simulink model "pvtest1"  (R2022b)
settings: Solver=ode45  StartTime=0.0  StopTime=100.0  RelTol=1e-3
values from neighbouring files (symbols this model uses):
  Ki1 = double(1)    [untitled.m]
  Ki2 = double(1)    [untitled.m]
  Kp1 = double(1)    [untitled.m]
  Kp2 = double(1)    [untitled.m]
undefined symbols (not defined in the file or in its folder): Kd1, Kd2, magnitude
libraries: slpidlib x2
settings Model: Creator=19693  LastModifiedBy=TT

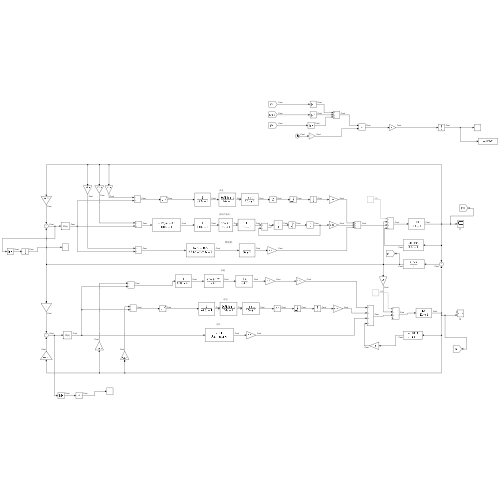
[thumbnail: Simulink's stored preview of the top-level diagram]
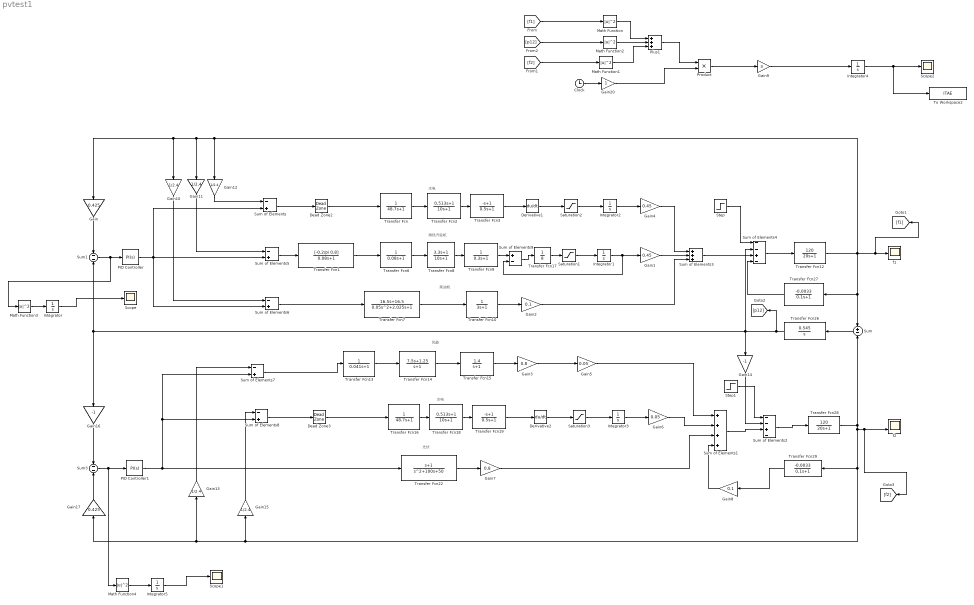
== system pvtest1 ==
  note: 光伏
  note: 风能
  note: 柴油机
  note: 再热汽轮机
  note: 水电
  note: 水电
  Clock : Clock
  Dead Zone2 : DeadZone  LowerValue=-0.0002  UpperValue=0.0002
  Dead Zone3 : DeadZone  LowerValue=-0.0002  UpperValue=0.0002
  Derivative1 : Derivative
  Derivative2 : Derivative
  Gain : Gain  Gain=0.425
  Gain1 : Gain  Gain=0.45
  Gain{10..13,15} (5 alike) : Gain  Gain=1/2.4
  Gain14 : Gain  Gain=-1
  Gain16 : Gain  Gain=-1
  Gain17 : Gain  Gain=0.425
  Gain2 : Gain  Gain=0.1
  Gain20 : Gain
  Gain3 : Gain  Gain=0.8
  Gain4 : Gain  Gain=0.45
  Gain5 : Gain  Gain=0.05
  Gain6 : Gain  Gain=0.05
  Gain7 : Gain  Gain=0.8
  Gain8 : Gain  Gain=0.1
  Gain9 : Gain  Gain=3
  Integrator{,1..5} (6 alike) : Integrator
  Math Function{,1..4} (5 alike) : Math  Operator=magnitude^2
  PID Controller : slpidlib/PID Controller  Controller=PI  Form=Parallel  TimeDomain=Continuous-time  UseExternalTs=off  SampleTime=-1  IntegratorMethod=Forward Euler  FilterMethod=Forward Euler  ControllerParametersSource=internal  P=Kp1  I=Ki1  UseKiTs=off  D=Kd1  N=100  UseFilter=on  TunerSelectOption=Transfer Function Based (PID Tuner App)  InitialConditionSource=internal  InitialConditionForIntegrator=0  InitialConditionForFilter=0  DifferentiatorICPrevScaledInput=0  ExternalReset=none  TrackingMode=off  Kt=1  LimitOutput=off  SatLimitsSource=internal  UpperSaturationLimit=inf  LowerSaturationLimit=-inf  LinearizeAsGain=on  AntiWindupMode=none  Kb=1  LimitIntegrator=off  UpperIntegratorSaturationLimit=inf  LowerIntegratorSaturationLimit=-inf  POutMin=[]  POutMax=[]  IOutMin=[]  IOutMax=[]  DOutMin=[]  DOutMax=[]  NOutMin=[]  NOutMax=[]  SumOutMin=[]  SumOutMax=[]  SaturationOutMin=[]  SaturationOutMax=[]  PParamMin=[]  PParamMax=[]  IParamMin=[]  IParamMax=[]  DParamMin=[]  DParamMax=[]  NParamMin=[]  NParamMax=[]  KbParamMin=[]  KbParamMax=[]  KtParamMin=[]  KtParamMax=[]  KbOutMin=[]  KbOutMax=[]  KtOutMin=[]  KtOutMax=[]  IntegratorOutMin=[]  IntegratorOutMax=[]  FilterOutMin=[]  FilterOutMax=[]  SumI1OutMin=[]  SumI1OutMax=[]  SumI2OutMin=[]  SumI2OutMax=[]  SumI3OutMin=[]  SumI3OutMax=[]  SumI4OutMin=[]  SumI4OutMax=[]  SumDOutMin=[]  SumDOutMax=[]  DifferentiatorOutMin=[]  DifferentiatorOutMax=[]  FilterDiffOutCoefMin=[]  FilterDiffOutCoefMax=[]  ReciprocalOutMin=[]  ReciprocalOutMax=[]  SumDenOutMin=[]  SumDenOutMax=[]  SumNumOutMin=[]  SumNumOutMax=[]  DivideOutMin=[]  DivideOutMax=[]  UdiffTsProdOutMin=[]  UdiffTsProdOutMax=[]  NTsProdOutMin=[]  NTsProdOutMax=[]  UintegralTsProdOutMin=[]  UintegralTsProdOutMax=[]  UngainTsProdOutMin=[]  UngainTsProdOutMax=[]  ClampingZeroOutDataTypeStr=Inherit: Inherit via back propagation  ClampingZeroOutMin=[]  ClampingZeroOutMax=[]  FilterDenConstantOutDataTypeStr=Inherit: Inherit via back propagation  FilterDenConstantOutMin=[]  FilterDenConstantOutMax=[]  PCopyOutDataTypeStr=Inherit: Inherit via back propagation  PCopyOutMin=[]  PCopyOutMax=[]  NCopyOutDataTypeStr=Inherit: Inherit via back propagation  NCopyOutMin=[]  NCopyOutMax=[]  IntegratorContinuousStateAttributes=''  IntegratorStateMustResolveToSignalObject=off  IntegratorRTWStateStorageClass=Auto  FilterContinuousStateAttributes=''  FilterStateMustResolveToSignalObject=off  FilterRTWStateStorageClass=Auto  ParallelPVariant=InternalParameters  IdealPVariant=Disabled  IVariant=InternalParameters  DVariant=Disabled  IntegratorVariant=Continuous  SatVariant=Disabled  AWVariant=Passthrough  PCopyVariant=Disabled  TRVariant=Disabled  FdbkBlocksVariant=Forward  IdealPFdbkVariant=Disabled  SatFdbkVariant=Disabled  DerivativeFilterVariant=Disabled  NVariant=Disabled  NCopyVariant=Disabled_SignalSpec  FilterICVariant=Disabled  IntegratorICVariant=InternalICs  ExternalResetVariant=Disabled  TRSumVariant=Passthrough  SumFdbkVariant=Disabled  SumVariant=Sum_PI  TsampFilterVariant=InternalTs  TsampNgainVariant=Passthrough  TsampIntegralVariant=Passthrough  ExternalSaturationOutDataTypeStr=Inherit: Same as second input
  PID Controller1 : slpidlib/PID Controller  Controller=PI  Form=Parallel  TimeDomain=Continuous-time  UseExternalTs=off  SampleTime=-1  IntegratorMethod=Forward Euler  FilterMethod=Forward Euler  ControllerParametersSource=internal  P=Kp2  I=Ki2  UseKiTs=off  D=Kd2  N=100  UseFilter=on  TunerSelectOption=Transfer Function Based (PID Tuner App)  InitialConditionSource=internal  InitialConditionForIntegrator=0  InitialConditionForFilter=0  DifferentiatorICPrevScaledInput=0  ExternalReset=none  TrackingMode=off  Kt=1  LimitOutput=off  SatLimitsSource=internal  UpperSaturationLimit=inf  LowerSaturationLimit=-inf  LinearizeAsGain=on  AntiWindupMode=none  Kb=1  LimitIntegrator=off  UpperIntegratorSaturationLimit=inf  LowerIntegratorSaturationLimit=-inf  POutMin=[]  POutMax=[]  IOutMin=[]  IOutMax=[]  DOutMin=[]  DOutMax=[]  NOutMin=[]  NOutMax=[]  SumOutMin=[]  SumOutMax=[]  SaturationOutMin=[]  SaturationOutMax=[]  PParamMin=[]  PParamMax=[]  IParamMin=[]  IParamMax=[]  DParamMin=[]  DParamMax=[]  NParamMin=[]  NParamMax=[]  KbParamMin=[]  KbParamMax=[]  KtParamMin=[]  KtParamMax=[]  KbOutMin=[]  KbOutMax=[]  KtOutMin=[]  KtOutMax=[]  IntegratorOutMin=[]  IntegratorOutMax=[]  FilterOutMin=[]  FilterOutMax=[]  SumI1OutMin=[]  SumI1OutMax=[]  SumI2OutMin=[]  SumI2OutMax=[]  SumI3OutMin=[]  SumI3OutMax=[]  SumI4OutMin=[]  SumI4OutMax=[]  SumDOutMin=[]  SumDOutMax=[]  DifferentiatorOutMin=[]  DifferentiatorOutMax=[]  FilterDiffOutCoefMin=[]  FilterDiffOutCoefMax=[]  ReciprocalOutMin=[]  ReciprocalOutMax=[]  SumDenOutMin=[]  SumDenOutMax=[]  SumNumOutMin=[]  SumNumOutMax=[]  DivideOutMin=[]  DivideOutMax=[]  UdiffTsProdOutMin=[]  UdiffTsProdOutMax=[]  NTsProdOutMin=[]  NTsProdOutMax=[]  UintegralTsProdOutMin=[]  UintegralTsProdOutMax=[]  UngainTsProdOutMin=[]  UngainTsProdOutMax=[]  ClampingZeroOutDataTypeStr=Inherit: Inherit via back propagation  ClampingZeroOutMin=[]  ClampingZeroOutMax=[]  FilterDenConstantOutDataTypeStr=Inherit: Inherit via back propagation  FilterDenConstantOutMin=[]  FilterDenConstantOutMax=[]  PCopyOutDataTypeStr=Inherit: Inherit via back propagation  PCopyOutMin=[]  PCopyOutMax=[]  NCopyOutDataTypeStr=Inherit: Inherit via back propagation  NCopyOutMin=[]  NCopyOutMax=[]  IntegratorContinuousStateAttributes=''  IntegratorStateMustResolveToSignalObject=off  IntegratorRTWStateStorageClass=Auto  FilterContinuousStateAttributes=''  FilterStateMustResolveToSignalObject=off  FilterRTWStateStorageClass=Auto  ParallelPVariant=InternalParameters  IdealPVariant=Disabled  IVariant=InternalParameters  DVariant=Disabled  IntegratorVariant=Continuous  SatVariant=Disabled  AWVariant=Passthrough  PCopyVariant=Disabled  TRVariant=Disabled  FdbkBlocksVariant=Forward  IdealPFdbkVariant=Disabled  SatFdbkVariant=Disabled  DerivativeFilterVariant=Disabled  NVariant=Disabled  NCopyVariant=Disabled_SignalSpec  FilterICVariant=Disabled  IntegratorICVariant=InternalICs  ExternalResetVariant=Disabled  TRSumVariant=Passthrough  SumFdbkVariant=Disabled  SumVariant=Sum_PI  TsampFilterVariant=InternalTs  TsampNgainVariant=Passthrough  TsampIntegralVariant=Passthrough  ExternalSaturationOutDataTypeStr=Inherit: Same as second input
  Plus1 : Sum  Inputs=+++
  Product : Product
  Saturation1 : Saturate
  Saturation2 : Saturate  UpperLimit=3.6  LowerLimit=-2.7
  Saturation3 : Saturate  UpperLimit=3.6  LowerLimit=-2.7
  Scope : Scope
  Scope1 : Scope
  Scope2 : Scope
  Step : Step  Time=0.01  After=0.05  SampleTime=0
  Step1 : Step  Time=0.01  After=0.05  SampleTime=0
  Sum : Sum  Inputs=+-
  Sum of Elements{,5..8} (5 alike) : Sum  Inputs=-+
  Sum of Elements1 : Sum  Inputs=++++
  Sum of Elements2 : Sum  Inputs=--+-
  Sum of Elements3 : Sum  Inputs=+++
  Sum of Elements4 : Sum  Inputs=--+-
  Sum of Elements9 : Sum  Inputs=+-
  Sum1 : Sum  Inputs=--
  Sum3 : Sum  Inputs=--
  To Workspace2 : ToWorkspace  VariableName=ITAE  SampleTime=-1
  Transfer Fcn : TransferFcn  Numerator=[0 1]  Denominator=[48.7 1]
  Transfer Fcn1 : TransferFcn  Numerator=[-0.2/pi 0.8]  Denominator=[0.08 1]
  Transfer Fcn10 : TransferFcn  Numerator=[0 1]  Denominator=[3 1]
  Transfer Fcn12 : TransferFcn  Numerator=[120]  Denominator=[20 1]
  Transfer Fcn13 : TransferFcn  Numerator=[0 1]  Denominator=[0.041 1]
  Transfer Fcn14 : TransferFcn  Numerator=[7.5 1.25]  Denominator=[1 1]
  Transfer Fcn15 : TransferFcn  Numerator=[1.4]  Denominator=[1 1]
  Transfer Fcn16 : TransferFcn  Numerator=[0 1]  Denominator=[48.7 1]
  Transfer Fcn17 : TransferFcn  Denominator=[8]
  Transfer Fcn18 : TransferFcn  Numerator=[0.513 1]  Denominator=[10 1]
  Transfer Fcn19 : TransferFcn  Numerator=[-1 1]  Denominator=[0.5 1]
  Transfer Fcn2 : TransferFcn  Numerator=[0.513 1]  Denominator=[10 1]
  Transfer Fcn22 : TransferFcn  Numerator=[1 1]  Denominator=[1 100 50]
  Transfer Fcn26 : TransferFcn  Numerator=[0.545]  Denominator=[1 0]
  Transfer Fcn27 : TransferFcn  Numerator=[-0.0033]  Denominator=[0.1 1]
  Transfer Fcn28 : TransferFcn  Numerator=[120]  Denominator=[20 1]
  Transfer Fcn29 : TransferFcn  Numerator=[-0.0033]  Denominator=[0.1 1]
  Transfer Fcn3 : TransferFcn  Numerator=[-1 1]  Denominator=[0.5 1]
  Transfer Fcn6 : TransferFcn  Numerator=[0 1]  Denominator=[0.08 1]
  Transfer Fcn7 : TransferFcn  Numerator=[16.5 16.5]  Denominator=[0.05 2.025 1]
  Transfer Fcn8 : TransferFcn  Numerator=[3.3 1]  Denominator=[10 1]
  Transfer Fcn9 : TransferFcn  Denominator=[0.3 1]
  f1 : Scope
      settings: Tag=f1
  f2 : Scope  NumInputPorts=2
      settings: Tag=f2
  wires:
  Transfer Fcn2/1 -> Transfer Fcn3/1
  Transfer Fcn/1 -> Transfer Fcn2/1
  Saturation1/1 -> Integrator1/1
  Transfer Fcn6/1 -> Transfer Fcn8/1
  Transfer Fcn8/1 -> Transfer Fcn9/1
  Transfer Fcn7/1 -> Transfer Fcn10/1
  Transfer Fcn10/1 -> Gain2/1
  Gain1/1 -> Sum of Elements3/2
  Gain4/1 -> Sum of Elements3/1
  Gain2/1 -> Sum of Elements3/3
  Sum of Elements3/1 -> Sum of Elements4/3
  Step/1 -> Sum of Elements4/1
  Sum of Elements4/1 -> Transfer Fcn12/1
  Transfer Fcn13/1 -> Transfer Fcn14/1
  Transfer Fcn14/1 -> Transfer Fcn15/1
  Transfer Fcn15/1 -> Gain3/1
  Gain3/1 -> Gain5/1
  Transfer Fcn16/1 -> Transfer Fcn18/1
  Transfer Fcn18/1 -> Transfer Fcn19/1
  Transfer Fcn22/1 -> Gain7/1
  Gain5/1 -> Sum of Elements1/1
  Gain6/1 -> Sum of Elements1/2
  Gain7/1 -> Sum of Elements1/3
  Sum of Elements1/1 -> Sum of Elements2/3
  Gain14/1 -> Sum of Elements2/2
  Sum/1 -> Transfer Fcn26/1
  Transfer Fcn26/1 -> Gain16/1, Sum1/2, Gain14/1, Sum of Elements4/2, [p12]
  Transfer Fcn27/1 -> Sum of Elements4/4
  Sum of Elements2/1 -> Transfer Fcn28/1
  Step1/1 -> Sum of Elements2/1
  Transfer Fcn12/1 -> Sum/1, Transfer Fcn27/1, [f1], f1/1, Gain12/1, Gain10/1, Gain/1, Gain11/1
  Gain12/1 -> Sum of Elements/1
  Gain11/1 -> Sum of Elements5/1
  Gain10/1 -> Sum of Elements6/1
  Sum of Elements/1 -> Dead Zone2/1
  Sum of Elements6/1 -> Transfer Fcn7/1
  Gain/1 -> Sum1/1
  Transfer Fcn28/1 -> [f2], f2/2, Transfer Fcn29/1, Gain17/1, Gain13/1, Gain15/1, Sum/2
  Gain13/1 -> Sum of Elements7/1
  Gain15/1 -> Sum of Elements8/1
  Gain16/1 -> Sum3/1
  Gain17/1 -> Sum3/2
  Sum of Elements7/1 -> Transfer Fcn13/1
  Dead Zone2/1 -> Transfer Fcn/1
  Sum of Elements5/1 -> Transfer Fcn1/1
  Transfer Fcn1/1 -> Transfer Fcn6/1
  Sum of Elements8/1 -> Dead Zone3/1
  Dead Zone3/1 -> Transfer Fcn16/1
  Transfer Fcn17/1 -> Saturation1/1
  Transfer Fcn9/1 -> Sum of Elements9/1
  Sum of Elements9/1 -> Transfer Fcn17/1
  Integrator1/1 -> Sum of Elements9/2, Gain1/1
  Derivative1/1 -> Saturation2/1
  Saturation2/1 -> Integrator2/1
  Transfer Fcn3/1 -> Derivative1/1
  Integrator2/1 -> Gain4/1
  Derivative2/1 -> Saturation3/1
  Saturation3/1 -> Integrator3/1
  Transfer Fcn19/1 -> Derivative2/1
  Integrator3/1 -> Gain6/1
  Transfer Fcn29/1 -> Gain8/1
  Plus1/1 -> Product/1
  Math Function/1 -> Plus1/1
  Math Function1/1 -> Plus1/3
  Clock/1 -> Gain20/1
  Gain20/1 -> Product/2
  Product/1 -> Gain9/1
  [f2] -> Math Function1/1
  [f1] -> Math Function/1
  Gain9/1 -> Integrator4/1
  Gain8/1 -> Sum of Elements1/4
  [p12] -> Math Function2/1
  Math Function2/1 -> Plus1/2
  Sum1/1 -> Math Function3/1, PID Controller/1
  PID Controller/1 -> Sum of Elements6/2, Sum of Elements/2, Sum of Elements5/2
  Sum3/1 -> Math Function4/1, PID Controller1/1
  PID Controller1/1 -> Sum of Elements7/2, Sum of Elements8/2, Transfer Fcn22/1
  Integrator4/1 -> To Workspace2/1, Scope2/1
  Math Function3/1 -> Integrator/1
  Integrator/1 -> Scope/1
  Math Function4/1 -> Integrator5/1
  Integrator5/1 -> Scope1/1
